simulink library "ssc_Probes_2012b_scopes_org"  (Simulink 10.0)
settings: Solver=ode45  StartTime=0.0  StopTime=10.0  RelTol=1e-3  EnableMultiTasking=on
libraries: fl_lib x42, nesl_utility x31, fl_ps_legacy_lib x1
(part 2 of 2)

== system ssc_Probes_2012b_scopes_org/Pneumatic/AbsPressure ==
  AbsPressure : Scope
  PS-S : nesl_utility/PS-Simulink Converter  PhysicalDomain=network_engine_domain  LeftPortType=input  RightPortType=output  SubClassName=ps_output  Unit=Pa  AffineConversion=off
  Pneumatic Absolute Reference : fl_lib/Pneumatic/Pneumatic Elements/Pneumatic Absolute Reference  G_Log=off  Q_Log=off  LocalVarNames=|G|Q  LocalVarDescs=|G|Q  LocalVarLogging=[0 0]
      settings: SourceProductName=Simscape  SourceProductBaseCode=SS
  Pneumatic Pressure & Temperature Sensor : fl_lib/Pneumatic/Pneumatic Sensors/Pneumatic Pressure & Temperature Sensor  pressure_difference_Log=off  gas_flow_Log=off  temperature_difference_Log=off  heat_flow_Log=off  LocalVarNames=|pressure_difference|gas_flow|temperature_difference|heat_flow  LocalVarDescs=|pressure_difference|gas_flow|temperature_difference|heat_flow  LocalVarLogging=[0 0 0 0]
      settings: SourceProductName=Simscape  SourceProductBaseCode=SS
  Terminator : Terminator
  A : PMIOPort  Side=Left
  wires:
  PS-S/1 -> [AbsPressure], AbsPressure/1  "AbsPressure"
  [AbsPressure] -> Terminator/1
  connections:
  A/RConn1 -- Pneumatic Pressure & Temperature Sensor/LConn1
  Pneumatic Absolute Reference/LConn1 -- Pneumatic Pressure & Temperature Sensor/RConn1
  PS-S/LConn1 -- Pneumatic Pressure & Temperature Sensor/RConn2

== system ssc_Probes_2012b_scopes_org/Pneumatic/AbsTemperature ==
  AbsTemperature : Scope
  PS-S : nesl_utility/PS-Simulink Converter  PhysicalDomain=network_engine_domain  LeftPortType=input  RightPortType=output  SubClassName=ps_output  Unit=K  AffineConversion=off
  Pneumatic Absolute Reference : fl_lib/Pneumatic/Pneumatic Elements/Pneumatic Absolute Reference  G_Log=off  Q_Log=off  LocalVarNames=|G|Q  LocalVarDescs=|G|Q  LocalVarLogging=[0 0]
      settings: SourceProductName=Simscape  SourceProductBaseCode=SS
  Pneumatic Pressure & Temperature Sensor : fl_lib/Pneumatic/Pneumatic Sensors/Pneumatic Pressure & Temperature Sensor  pressure_difference_Log=off  gas_flow_Log=off  temperature_difference_Log=off  heat_flow_Log=off  LocalVarNames=|pressure_difference|gas_flow|temperature_difference|heat_flow  LocalVarDescs=|pressure_difference|gas_flow|temperature_difference|heat_flow  LocalVarLogging=[0 0 0 0]
      settings: SourceProductName=Simscape  SourceProductBaseCode=SS
  Terminator : Terminator
  A : PMIOPort  Side=Left
  wires:
  PS-S/1 -> AbsTemperature/1, [AbsTemperature]  "AbsTemperature"
  [AbsTemperature] -> Terminator/1
  connections:
  PS-S/LConn1 -- Pneumatic Pressure & Temperature Sensor/RConn3
  Pneumatic Absolute Reference/LConn1 -- Pneumatic Pressure & Temperature Sensor/RConn1
  A/RConn1 -- Pneumatic Pressure & Temperature Sensor/LConn1

== system ssc_Probes_2012b_scopes_org/Pneumatic/AtmTemperature ==
  AtmTemperature : Scope
  PS-S : nesl_utility/PS-Simulink Converter  PhysicalDomain=network_engine_domain  LeftPortType=input  RightPortType=output  SubClassName=ps_output  Unit=K  AffineConversion=off
  Pneumatic Atmospheric Reference : fl_lib/Pneumatic/Pneumatic Elements/Pneumatic Atmospheric Reference  gas_flow_Log=off  heat_flow_Log=off  LocalVarNames=|gas_flow|heat_flow  LocalVarDescs=|gas_flow|heat_flow  LocalVarLogging=[0 0]
      settings: SourceProductName=Simscape  SourceProductBaseCode=SS
  Pneumatic Pressure & Temperature Sensor : fl_lib/Pneumatic/Pneumatic Sensors/Pneumatic Pressure & Temperature Sensor  pressure_difference_Log=off  gas_flow_Log=off  temperature_difference_Log=off  heat_flow_Log=off  LocalVarNames=|pressure_difference|gas_flow|temperature_difference|heat_flow  LocalVarDescs=|pressure_difference|gas_flow|temperature_difference|heat_flow  LocalVarLogging=[0 0 0 0]
      settings: SourceProductName=Simscape  SourceProductBaseCode=SS
  Terminator : Terminator
  A : PMIOPort  Side=Left
  wires:
  PS-S/1 -> AtmTemperature/1, [AtmTemperature]  "AtmTemperature"
  [AtmTemperature] -> Terminator/1
  connections:
  A/RConn1 -- Pneumatic Pressure & Temperature Sensor/LConn1
  Pneumatic Atmospheric Reference/LConn1 -- Pneumatic Pressure & Temperature Sensor/RConn1
  PS-S/LConn1 -- Pneumatic Pressure & Temperature Sensor/RConn3

== system ssc_Probes_2012b_scopes_org/Pneumatic/GasHeatFlow ==
  GasHeatFlow : Scope
  PS-S : nesl_utility/PS-Simulink Converter  PhysicalDomain=network_engine_domain  LeftPortType=input  RightPortType=output  SubClassName=ps_output  Unit=J/s  AffineConversion=off
  Pneumatic Mass & Heat Flow Sensor : fl_lib/Pneumatic/Pneumatic Sensors/Pneumatic Mass & Heat Flow Sensor  pressure_difference_Log=off  gas_flow_Log=off  temperature_difference_Log=off  heat_flow_Log=off  LocalVarNames=|pressure_difference|gas_flow|temperature_difference|heat_flow  LocalVarDescs=|pressure_difference|gas_flow|temperature_difference|heat_flow  LocalVarLogging=[0 0 0 0]
      settings: SourceProductName=Simscape  SourceProductBaseCode=SS
  Terminator : Terminator
  A : PMIOPort  Side=Left
  B : PMIOPort  Port=2  Side=Right
  wires:
  PS-S/1 -> GasHeatFlow/1, [GasHeatFlow]  "GasHeatFlow"
  [GasHeatFlow] -> Terminator/1
  connections:
  PS-S/LConn1 -- Pneumatic Mass & Heat Flow Sensor/RConn3
  B/RConn1 -- Pneumatic Mass & Heat Flow Sensor/RConn1
  A/RConn1 -- Pneumatic Mass & Heat Flow Sensor/LConn1

== system ssc_Probes_2012b_scopes_org/Pneumatic/GaugePressure ==
  GaugePressure : Scope
  PS-S : nesl_utility/PS-Simulink Converter  PhysicalDomain=network_engine_domain  LeftPortType=input  RightPortType=output  SubClassName=ps_output  Unit=Pa  AffineConversion=off
  Pneumatic Atmospheric Reference : fl_lib/Pneumatic/Pneumatic Elements/Pneumatic Atmospheric Reference  gas_flow_Log=off  heat_flow_Log=off  LocalVarNames=|gas_flow|heat_flow  LocalVarDescs=|gas_flow|heat_flow  LocalVarLogging=[0 0]
      settings: SourceProductName=Simscape  SourceProductBaseCode=SS
  Pneumatic Pressure & Temperature Sensor : fl_lib/Pneumatic/Pneumatic Sensors/Pneumatic Pressure & Temperature Sensor  pressure_difference_Log=off  gas_flow_Log=off  temperature_difference_Log=off  heat_flow_Log=off  LocalVarNames=|pressure_difference|gas_flow|temperature_difference|heat_flow  LocalVarDescs=|pressure_difference|gas_flow|temperature_difference|heat_flow  LocalVarLogging=[0 0 0 0]
      settings: SourceProductName=Simscape  SourceProductBaseCode=SS
  Terminator : Terminator
  A : PMIOPort  Side=Left
  wires:
  PS-S/1 -> GaugePressure/1, [GaugePressure]  "GaugePressure"
  [GaugePressure] -> Terminator/1
  connections:
  PS-S/LConn1 -- Pneumatic Pressure & Temperature Sensor/RConn2
  Pneumatic Atmospheric Reference/LConn1 -- Pneumatic Pressure & Temperature Sensor/RConn1
  A/RConn1 -- Pneumatic Pressure & Temperature Sensor/LConn1

== system ssc_Probes_2012b_scopes_org/Pneumatic/MassFlow ==
  MassFlow : Scope
  PS-S : nesl_utility/PS-Simulink Converter  PhysicalDomain=network_engine_domain  LeftPortType=input  RightPortType=output  SubClassName=ps_output  Unit=kg/s  AffineConversion=off
  Pneumatic Mass & Heat Flow Sensor : fl_lib/Pneumatic/Pneumatic Sensors/Pneumatic Mass & Heat Flow Sensor  pressure_difference_Log=off  gas_flow_Log=off  temperature_difference_Log=off  heat_flow_Log=off  LocalVarNames=|pressure_difference|gas_flow|temperature_difference|heat_flow  LocalVarDescs=|pressure_difference|gas_flow|temperature_difference|heat_flow  LocalVarLogging=[0 0 0 0]
      settings: SourceProductName=Simscape  SourceProductBaseCode=SS
  Terminator : Terminator
  A : PMIOPort  Side=Left
  B : PMIOPort  Port=2  Side=Right
  wires:
  PS-S/1 -> [MassFlow], MassFlow/1  "MassFlow"
  [MassFlow] -> Terminator/1
  connections:
  A/RConn1 -- Pneumatic Mass & Heat Flow Sensor/LConn1
  Pneumatic Mass & Heat Flow Sensor/RConn2 -- PS-S/LConn1
  B/RConn1 -- Pneumatic Mass & Heat Flow Sensor/RConn1

== system ssc_Probes_2012b_scopes_org/Pneumatic/dGasPressure ==
  GasPressure : Scope
  PS-S : nesl_utility/PS-Simulink Converter  PhysicalDomain=network_engine_domain  LeftPortType=input  RightPortType=output  SubClassName=ps_output  Unit=Pa  AffineConversion=off
  Pneumatic Pressure & Temperature Sensor : fl_lib/Pneumatic/Pneumatic Sensors/Pneumatic Pressure & Temperature Sensor  pressure_difference_Log=off  gas_flow_Log=off  temperature_difference_Log=off  heat_flow_Log=off  LocalVarNames=|pressure_difference|gas_flow|temperature_difference|heat_flow  LocalVarDescs=|pressure_difference|gas_flow|temperature_difference|heat_flow  LocalVarLogging=[0 0 0 0]
      settings: SourceProductName=Simscape  SourceProductBaseCode=SS
  Terminator : Terminator
  A : PMIOPort  Side=Left
  B : PMIOPort  Port=2  Side=Right
  wires:
  PS-S/1 -> [dGasPressure], GasPressure/1  "GasPressure"
  [dGasPressure] -> Terminator/1
  connections:
  A/RConn1 -- Pneumatic Pressure & Temperature Sensor/LConn1
  B/RConn1 -- Pneumatic Pressure & Temperature Sensor/RConn1
  Pneumatic Pressure & Temperature Sensor/RConn2 -- PS-S/LConn1

== system ssc_Probes_2012b_scopes_org/Pneumatic/dGasTemperature ==
  PS-S : nesl_utility/PS-Simulink Converter  PhysicalDomain=network_engine_domain  LeftPortType=input  RightPortType=output  SubClassName=ps_output  Unit=K  AffineConversion=off
  Pneumatic Pressure & Temperature Sensor : fl_lib/Pneumatic/Pneumatic Sensors/Pneumatic Pressure & Temperature Sensor  pressure_difference_Log=off  gas_flow_Log=off  temperature_difference_Log=off  heat_flow_Log=off  LocalVarNames=|pressure_difference|gas_flow|temperature_difference|heat_flow  LocalVarDescs=|pressure_difference|gas_flow|temperature_difference|heat_flow  LocalVarLogging=[0 0 0 0]
      settings: SourceProductName=Simscape  SourceProductBaseCode=SS
  Terminator : Terminator
  dGasTemperature : Scope
  A : PMIOPort  Side=Left
  B : PMIOPort  Port=2  Side=Right
  wires:
  PS-S/1 -> dGasTemperature/1, [dGasTemperature]  "dGasTemperaature"
  [dGasTemperature] -> Terminator/1
  connections:
  PS-S/LConn1 -- Pneumatic Pressure & Temperature Sensor/RConn3
  B/RConn1 -- Pneumatic Pressure & Temperature Sensor/RConn1
  A/RConn1 -- Pneumatic Pressure & Temperature Sensor/LConn1

== system ssc_Probes_2012b_scopes_org/Thermal/HeatFlow ==
  Ideal Heat Flow Sensor : fl_lib/Thermal/Thermal Sensors/Ideal Heat Flow Sensor  Q_Log=off  T_Log=off  LocalVarNames=|Q|T  LocalVarDescs=|Q|T  LocalVarLogging=[]
      settings: SourceProductName=Simscape  SourceProductBaseCode=SS
  PS-S : nesl_utility/PS-Simulink Converter  PhysicalDomain=network_engine_domain  LeftPortType=input  RightPortType=output  SubClassName=ps_output  Unit=J/s  AffineConversion=off
  Terminator : Terminator
  heat flow : Scope
  A : PMIOPort  Side=Left
  B : PMIOPort  Port=2  Side=Right
  wires:
  PS-S/1 -> heat flow/1, [HeatFlow]  "heat flow"
  [HeatFlow] -> Terminator/1
  connections:
  A/RConn1 -- Ideal Heat Flow Sensor/LConn1
  Ideal Heat Flow Sensor/RConn1 -- PS-S/LConn1
  B/RConn1 -- Ideal Heat Flow Sensor/RConn2

== system ssc_Probes_2012b_scopes_org/Thermal/Temperature ==
  Ideal Temperature Sensor : fl_lib/Thermal/Thermal Sensors/Ideal Temperature Sensor  Qs_Log=off  Ts_Log=off  LocalVarNames=|Qs|Ts  LocalVarDescs=|Qs|Ts  LocalVarLogging=[]
      settings: SourceProductName=Simscape  SourceProductBaseCode=SS
  PS-S : nesl_utility/PS-Simulink Converter  PhysicalDomain=network_engine_domain  LeftPortType=input  RightPortType=output  SubClassName=ps_output  Unit=K  AffineConversion=off
  Terminator : Terminator
  Thermal Reference : fl_lib/Thermal/Thermal Elements/Thermal Reference  Q_Log=off  LocalVarNames=|Q  LocalVarDescs=|Q  LocalVarLogging=0
  temperature : Scope
  A : PMIOPort  Side=Left
  wires:
  PS-S/1 -> temperature/1, [Temperature]  "temperature"
  [Temperature] -> Terminator/1
  connections:
  A/RConn1 -- Ideal Temperature Sensor/LConn1
  Thermal Reference/LConn1 -- Ideal Temperature Sensor/RConn1
  PS-S/LConn1 -- Ideal Temperature Sensor/RConn2

== system ssc_Probes_2012b_scopes_org/Thermal/dTemperature ==
  Ideal Temperature Sensor : fl_lib/Thermal/Thermal Sensors/Ideal Temperature Sensor  Qs_Log=off  Ts_Log=off  LocalVarNames=|Qs|Ts  LocalVarDescs=|Qs|Ts  LocalVarLogging=[]
      settings: SourceProductName=Simscape  SourceProductBaseCode=SS
  PS-S : nesl_utility/PS-Simulink Converter  PhysicalDomain=network_engine_domain  LeftPortType=input  RightPortType=output  SubClassName=ps_output  Unit=K  AffineConversion=off
  Terminator : Terminator
  temperature : Scope
  A : PMIOPort  Side=Left
  B : PMIOPort  Port=2  Side=Right
  wires:
  PS-S/1 -> temperature/1, [dTemperature]  "temperature"
  [dTemperature] -> Terminator/1
  connections:
  PS-S/LConn1 -- Ideal Temperature Sensor/RConn2
  B/RConn1 -- Ideal Temperature Sensor/RConn1
  A/RConn1 -- Ideal Temperature Sensor/LConn1
